simulink model "modelo_robot_3dof_dindir"  (R2023b)
settings: Solver=ode45  StartTime=0.0  StopTime=tsim  MaxStep=1e-2  RelTol=1e-3
undefined symbols (not defined in the file): robot_params, tau_L, tau_Rref
settings Model: Creator=HP  LastModifiedBy=HP

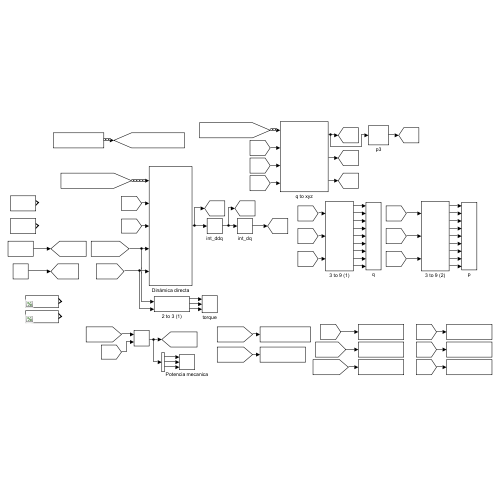
[thumbnail: Simulink's stored preview of the top-level diagram]
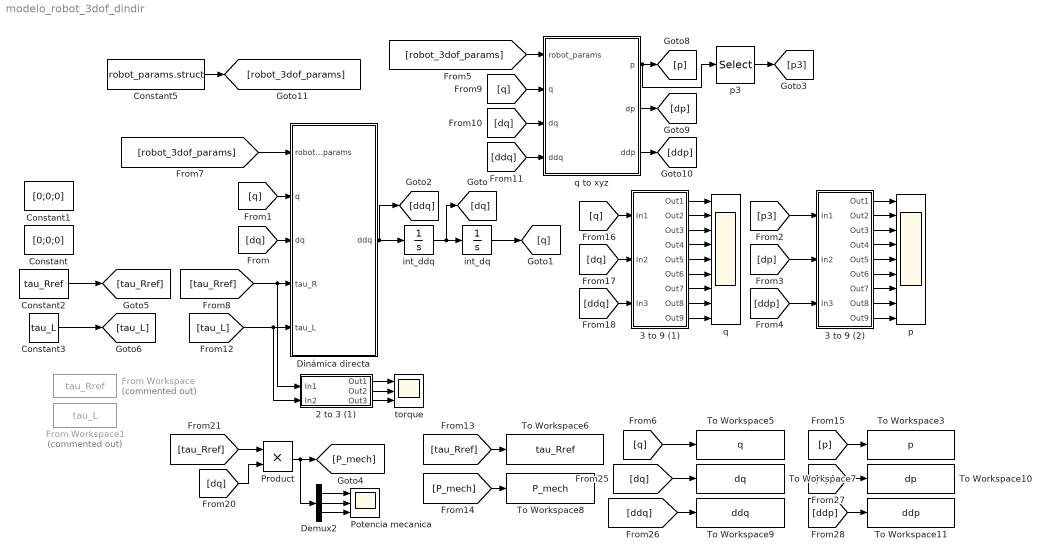
== system modelo_robot_3dof_dindir ==
  2 to 3 (1) : Subsystem
  3 to 9 (1) : Subsystem
  3 to 9 (2) : Subsystem
  Constant : Constant  Value=[0;0;0]
  Constant1 : Constant  Value=[0;0;0]
  Constant2 : Constant  Value=tau_Rref
  Constant3 : Constant  Value=tau_L
  Constant5 : Constant  Value=robot_params.struct  OutDataTypeStr=Bus: robot_params_bus
  Demux2 : Demux  Outputs=3
  Dinámica directa : MATLAB Function  TreatAsAtomicUnit=on
  From Workspace : FromWorkspace  Commented=on  VariableName=tau_Rref
  From Workspace1 : FromWorkspace  Commented=on  VariableName=tau_L
  Potencia mecanica : Scope  NumInputPorts=3
  Product : Product
  To Workspace10 : ToWorkspace  VariableName=dp  SaveFormat=Timeseries  SampleTime=-1
  To Workspace11 : ToWorkspace  VariableName=ddp  SaveFormat=Timeseries  SampleTime=-1
  To Workspace3 : ToWorkspace  VariableName=p  SaveFormat=Timeseries  SampleTime=-1
  To Workspace5 : ToWorkspace  VariableName=q  SaveFormat=Timeseries  SampleTime=-1
  To Workspace6 : ToWorkspace  VariableName=tau_Rref  SaveFormat=Timeseries  SampleTime=-1
  To Workspace7 : ToWorkspace  VariableName=dq  SaveFormat=Timeseries  SampleTime=-1
  To Workspace8 : ToWorkspace  VariableName=P_mech  SaveFormat=Timeseries  SampleTime=-1
  To Workspace9 : ToWorkspace  VariableName=ddq  SaveFormat=Timeseries  SampleTime=-1
  int_ddq : Integrator  InitialCondition=[0;0;0]
  int_dq : Integrator  InitialCondition=[0;-1.669;0]
  p : Scope  NumInputPorts=9
  p3 : Selector  NumberOfDimensions=2  InputPortWidth=3  IndexOptions=Index vector (dialog),Index vector (dialog)  Indices=[1:3],3  OutputSizes=1,1
  q : Scope  NumInputPorts=9
  q to xyz : MATLAB Function  TreatAsAtomicUnit=on
  torque : Scope  NumInputPorts=3
  wires:
  Dinámica directa/1(ddq) -> [ddq], int_ddq/1
  int_ddq/1 -> [dq], int_dq/1
  int_dq/1 -> [q]
  [dq] -> Dinámica directa/3(dq)
  [q] -> Dinámica directa/2(q)
  [tau_L] -> 2 to 3 (1)/2(In2), Dinámica directa/5(tau_L)
  Constant5/1 -> [robot_3dof_params]
  [robot_3dof_params] -> Dinámica directa/1(robot_params)
  [tau_Rref] -> 2 to 3 (1)/1(In1), Dinámica directa/4(tau_R)
  3 to 9 (1)/7(Out7) -> q/7
  3 to 9 (1)/9(Out9) -> q/9
  3 to 9 (1)/8(Out8) -> q/8
  3 to 9 (1)/2(Out2) -> q/2
  3 to 9 (1)/4(Out4) -> q/4
  3 to 9 (1)/5(Out5) -> q/5
  3 to 9 (1)/6(Out6) -> q/6
  3 to 9 (1)/1(Out1) -> q/1
  3 to 9 (1)/3(Out3) -> q/3
  [ddq] -> 3 to 9 (1)/3(In3)
  [q] -> 3 to 9 (1)/1(In1)
  [dq] -> 3 to 9 (1)/2(In2)
  [ddq] -> q to xyz/4(ddq)
  q to xyz/1(p) -> p3/1, [p]
  q to xyz/3(ddp) -> [ddp]
  [dq] -> q to xyz/3(dq)
  [q] -> q to xyz/2(q)
  [robot_3dof_params] -> q to xyz/1(robot_params)
  q to xyz/2(dp) -> [dp]
  2 to 3 (1)/1(Out1) -> torque/1
  3 to 9 (2)/9(Out9) -> p/9
  3 to 9 (2)/7(Out7) -> p/7
  [dp] -> 3 to 9 (2)/2(In2)
  [ddp] -> 3 to 9 (2)/3(In3)
  3 to 9 (2)/8(Out8) -> p/8
  3 to 9 (2)/1(Out1) -> p/1
  3 to 9 (2)/5(Out5) -> p/5
  3 to 9 (2)/6(Out6) -> p/6
  3 to 9 (2)/4(Out4) -> p/4
  3 to 9 (2)/3(Out3) -> p/3
  3 to 9 (2)/2(Out2) -> p/2
  p3/1 -> [p3]
  [p3] -> 3 to 9 (2)/1(In1)
  2 to 3 (1)/2(Out2) -> torque/2
  2 to 3 (1)/3(Out3) -> torque/3
  Demux2/3 -> Potencia mecanica/3
  Demux2/2 -> Potencia mecanica/2
  Product/1 -> Demux2/1, [P_mech]
  [dq] -> Product/2
  [tau_Rref] -> Product/1
  Demux2/1 -> Potencia mecanica/1
  Constant2/1 -> [tau_Rref]
  Constant3/1 -> [tau_L]
  [ddq] -> To Workspace9/1
  [P_mech] -> To Workspace8/1
  [dq] -> To Workspace7/1
  [q] -> To Workspace5/1
  [tau_Rref] -> To Workspace6/1
  [dp] -> To Workspace10/1
  [ddp] -> To Workspace11/1
  [p] -> To Workspace3/1

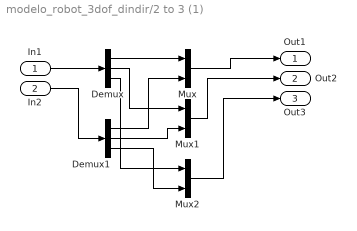
== system modelo_robot_3dof_dindir/2 to 3 (1) ==
  In1 : Inport
  In2 : Inport  Port=2
  Demux : Demux  Outputs=3
  Demux1 : Demux  Outputs=3
  Mux : Mux  Inputs=2
  Mux1 : Mux  Inputs=2
  Mux2 : Mux  Inputs=2
  Out1 : Outport
  Out2 : Outport  Port=2
  Out3 : Outport  Port=3
  wires:
  Demux/3 -> Mux2/1
  Mux2/1 -> Out3/1
  Mux1/1 -> Out2/1
  Demux/1 -> Mux/1
  Demux1/1 -> Mux/2
  In1/1 -> Demux/1
  Demux/2 -> Mux1/1
  Demux1/2 -> Mux1/2
  Mux/1 -> Out1/1
  Demux1/3 -> Mux2/2
  In2/1 -> Demux1/1

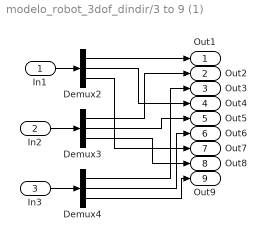
== system modelo_robot_3dof_dindir/3 to 9 (1) ==
  In1 : Inport
  In2 : Inport  Port=2
  In3 : Inport  Port=3
  Demux2 : Demux  Outputs=3
  Demux3 : Demux  Outputs=3
  Demux4 : Demux  Outputs=3
  Out1 : Outport
  Out2 : Outport  Port=2
  Out3 : Outport  Port=3
  Out4 : Outport  Port=4
  Out5 : Outport  Port=5
  Out6 : Outport  Port=6
  Out7 : Outport  Port=7
  Out8 : Outport  Port=8
  Out9 : Outport  Port=9
  wires:
  In3/1 -> Demux4/1
  Demux4/1 -> Out3/1
  Demux2/1 -> Out1/1
  Demux3/3 -> Out8/1
  Demux3/2 -> Out5/1
  Demux3/1 -> Out2/1
  In1/1 -> Demux2/1
  Demux2/3 -> Out7/1
  Demux4/3 -> Out9/1
  Demux4/2 -> Out6/1
  Demux2/2 -> Out4/1
  In2/1 -> Demux3/1

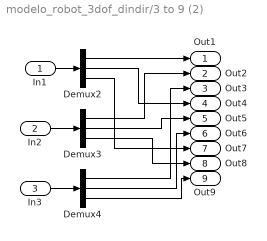
== system modelo_robot_3dof_dindir/3 to 9 (2) ==
  In1 : Inport
  In2 : Inport  Port=2
  In3 : Inport  Port=3
  Demux2 : Demux  Outputs=3
  Demux3 : Demux  Outputs=3
  Demux4 : Demux  Outputs=3
  Out1 : Outport
  Out2 : Outport  Port=2
  Out3 : Outport  Port=3
  Out4 : Outport  Port=4
  Out5 : Outport  Port=5
  Out6 : Outport  Port=6
  Out7 : Outport  Port=7
  Out8 : Outport  Port=8
  Out9 : Outport  Port=9
  wires:
  In3/1 -> Demux4/1
  Demux4/1 -> Out3/1
  Demux2/1 -> Out1/1
  Demux3/3 -> Out8/1
  Demux3/2 -> Out5/1
  Demux3/1 -> Out2/1
  In1/1 -> Demux2/1
  Demux2/3 -> Out7/1
  Demux4/3 -> Out9/1
  Demux4/2 -> Out6/1
  Demux2/2 -> Out4/1
  In2/1 -> Demux3/1

== matlab function modelo_robot_3dof_dindir/Dinámica directa ==
  data: robot_params input; q input size=[3,1]; ddq output size=[3,1]; dq input size=[3,1]; tau_R input size=[3,1]; tau_L input size=[3,1]
function ddq = fcn(robot_params,q,dq,tau_R,tau_L)

%d1 = robot_params.d(1);
l2 = robot_params.l(2);
lc2 = robot_params.lc(2);
%l3 = robot_params.l(3);
lc3 = robot_params.lc(3);

%m1 = robot_params.m(1);
m2 = robot_params.m(2);
m3 = robot_params.m(3);

Iz1 = robot_params.I(1,3);
Iy2 = robot_params.I(2,2);
Iz2 = robot_params.I(2,3);
Iy3 = robot_params.I(3,2);
Iz3 = robot_params.I(3,3);

g = 9.81;

q1 = q(1);
q2 = q(2);
q3 = q(3);

dq1 = dq(1);
dq2 = dq(2);
dq3 = dq(3);

D = zeros(3,3);

D(1,1) = Iz1 + Iz2 + Iz3 + (m2/2)*lc2^2*(1+cos(2*q2)) ...
       + (m3/2)*(l2^2*(1+cos(2*q2)) + 2*l2*lc3*(cos(2*q2+q3)+cos(q3)) ...
       + lc3^2*(1+cos(2*q2+2*q3)));

D(2,2) = Iy2 + Iy3 + m2*lc2^2 + m3*(l2^2 + 2*l2*lc3*cos(q3) + lc3^2);
D(2,3) = Iy3 + m3*(l2*lc3*cos(q3) + lc3^2);

D(3,2) = Iy3 + m3*(l2*lc3*cos(q3) + lc3^2);
D(3,3) = Iy3 + m3*lc3^2;

C = zeros(3,3);

C(1,2) = - ((m2*lc2^2*sin(2*q2)) ...
         + m3*(l2^2*sin(2*q2) + 2*l2*lc3*sin(2*q2+q3) ...
         + lc3^2*sin(2*q2+2*q3)))*dq1;
C(1,3) = - m3*(l2*lc3*(sin(2*q2+q3)+sin(q3)) ...
         + lc3^2*(sin(2*q2+2*q3)))*dq1;

C(2,1) =   ((m2/2)*(lc2^2*sin(2*q2)) ...
         + (m3/2)*(l2^2*sin(2*q2) + 2*l2*lc3*sin(2*q2+q3) ...
         + lc3^2*sin(2*q2+2*q3)))*dq1;
C(2,2) = - 2*m3*l2*lc3*sin(q3)*dq3;
C(2,3) = - m3*l2*lc3*sin(q3)*dq3;

C(3,1) =   (m3/2)*(l2*lc3*(sin(2*q2+q3) + sin(q3)) ...
         + lc3^2*sin(2*q2+2*q3))*dq1;
C(3,2) =   m3*l2*lc3*sin(q3)*dq2;

G = zeros(3,1);

G(2,1) = m2*lc2*cos(q2) + m3*(l2*cos(q2) + lc3*cos(q2+q3));
G(3,1) = m3*lc3*cos(q2+q3);



ddq = D^-1*(-C*dq-G*g+(tau_R-tau_L));

== matlab function modelo_robot_3dof_dindir/q to xyz ==
  data: robot_params input; p output size=[3,3]; q input size=[3,1]; dq input size=[3,1]; ddq input size=[3,1]; dp output size=[3,1]; ddp output size=[3,1]
function [p,dp,ddp] = fcn(robot_params,q,dq,ddq)

d1 = robot_params.d(1);
l2 = robot_params.l(2);
l3 = robot_params.l(3);

q1 = q(1);
q2 = q(2);
q3 = q(3);

p1 = [0;0;d1];

p2 = [l2*cos(q1)*cos(q2);
      l2*sin(q1)*cos(q2);
      d1+l2*sin(q2)];

p3 = [cos(q1)*(l2*cos(q2)+l3*cos(q2+q3));
      sin(q1)*(l2*cos(q2)+l3*cos(q2+q3));
      d1+l2*sin(q2)+l3*sin(q2+q3)];

p = [p1,p2,p3];

JP = zeros(3,3);

JP(1,1) = -sin(q1)*(l2*cos(q2) + l3*cos(q2 + q3));
JP(1,2) = -cos(q1)*(l2*sin(q2) + l3*sin(q2 + q3));
JP(1,3) = -l3*cos(q1)*sin(q2 + q3);

JP(2,1) =  cos(q1)*(l2*cos(q2) + l3*cos(q2 + q3));
JP(2,2) = -sin(q1)*(l2*sin(q2) + l3*sin(q2 + q3));
JP(2,3) = -l3*sin(q1)*sin(q2 + q3);

JP(3,2) = l2*cos(q2) + l3*cos(q2 + q3);
JP(3,3) = l3*cos(q2 + q3);

dp = JP*dq;
dq1 = dq(1);
dq2 = dq(2);
dq3 = dq(3);

dJ = zeros(3,3);

dJ(1,1) = - cos(q1)*(l2*cos(q2) + l3*cos(q2 + q3))*dq1 + sin(q1)*(l2*sin(q2) + l3*sin(q2 + q3))*dq2 + l3*sin(q1)*sin(q2 + q3)*dq3;
dJ(1,2) =   sin(q1)*(l2*sin(q2) + l3*sin(q2 + q3))*dq1 - cos(q1)*(l2*cos(q2) + l3*cos(q2 + q3))*dq2 - l3*cos(q1)*cos(q2 + q3)*dq3;
dJ(1,3) =   l3*sin(q1)*sin(q2 + q3)*dq1 - l3*cos(q1)*cos(q2 + q3)*dq2 - l3*cos(q1)*cos(q2 + q3)*dq3;

dJ(2,1) = - sin(q1)*(l2*cos(q2) + l3*cos(q2 + q3))*dq1 - cos(q1)*(l2*sin(q2) + l3*sin(q2 + q3))*dq2 - l3*cos(q1)*sin(q2 + q3)*dq3;
dJ(2,2) = - cos(q1)*(l2*sin(q2) + l3*sin(q2 + q3))*dq1 - sin(q1)*(l2*cos(q2) + l3*cos(q2 + q3))*dq2 - l3*sin(q1)*cos(q2 + q3)*dq3;
dJ(2,3) = - l3*cos(q1)*sin(q2 + q3)*dq1 - l3*sin(q1)*cos(q2 + q3)*dq2 - l3*sin(q1)*cos(q2 + q3)*dq3;

dJ(3,1) = 0;
dJ(3,2) = - (l2*sin(q2) + l3*sin(q2 + q3))*dq2 - l3*sin(q2 + q3)*dq3;
dJ(3,3) = - l3*sin(q2 + q3)*(dq2 + dq3);

ddp = dJ*ddq;
